simulink model "DC_motor"  (R2021b)
settings: Solver=VariableStepAuto  StartTime=0.0  StopTime=10.0  RelTol=1e-3
values from neighbouring files (symbols this model uses):
  Cmax = 0.66    [DC_moteur.sldd]
  Imax = 10.0    [DC_moteur.sldd]
  Ke = 0.041    [DC_moteur.sldd]
  Kt = 0.06    [DC_moteur.sldd]
  L = 0.00074    [DC_moteur.sldd]
  N1 = 4.25    [DC_moteur.sldd]
  R = 0.3    [DC_moteur.sldd]
  SigI = 0.05    [DC_moteur.sldd]
  Tech_Current = 0.01    [DC_moteur.sldd]
  vf_mot = 0.0    [DC_moteur.sldd]
libraries: simulink x1
settings Model: DataDictionary=DC_moteur.sldd  EnableAccessToBaseWorkspace=off  Creator=hugo  LastModifiedBy=hugo
settings SolverCC: ZeroCrossAlgorithm=Adaptive  AlgebraicLoopSolver=TrustRegion
settings DataIOCC: ReturnWorkspaceOutputs=off
settings DebuggingCC: SFMachineParentedDataDiag=warning  ArithmeticOperatorsInVariantConditions=warning
settings ModelReferenceCC: ModelReferenceMinAlgLoopOccurrences=on
settings SFSimCC: SimUseLocalCustomCode=off  CustomCodeUndefinedFunction=UseInterfaceOnly
settings RTWCC: RTWUseLocalCustomCode=off

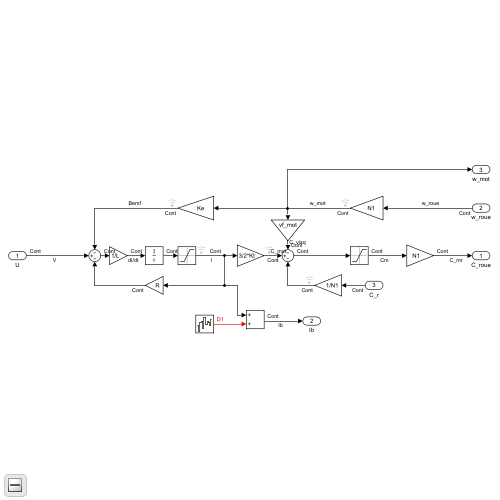
[thumbnail: Simulink's stored preview of the top-level diagram]
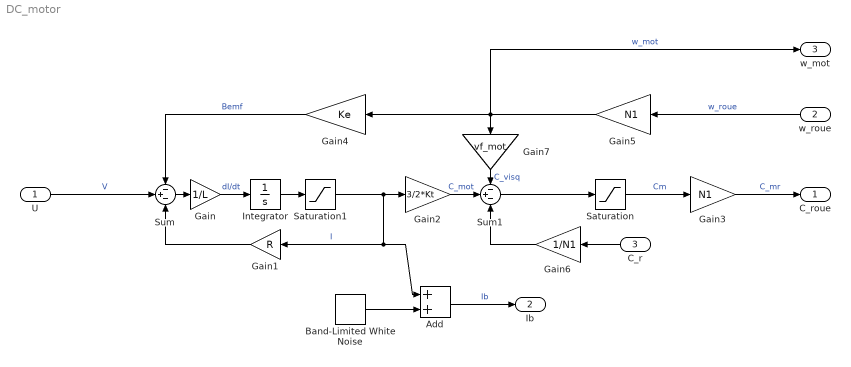
== system DC_motor ==
  U : Inport
  w_roue : Inport  Port=2
  C_r : Inport  Port=3
  Add : Sum
  Band-Limited White Noise : simulink/Sources/Band-Limited White Noise  Cov=(SigI)^2/(Tech_Current/2)  Ts=Tech_Current/2  seed=[23341]
  Gain : Gain  Gain=1/L
  Gain1 : Gain  Gain=R
  Gain2 : Gain  Gain=3/2*Kt
  Gain3 : Gain  Gain=N1
  Gain4 : Gain  Gain=Ke
  Gain5 : Gain  Gain=N1
  Gain6 : Gain  Gain=1/N1
  Gain7 : Gain  Gain=vf_mot
  Integrator : Integrator  ContinuousStateAttributes='Courant_Moteur'
  Saturation : Saturate  UpperLimit=Cmax  LowerLimit=-Cmax
  Saturation1 : Saturate  UpperLimit=Imax  LowerLimit=-Imax
  Sum : Sum  Inputs=-+-
  Sum1 : Sum  Inputs=-+-
  C_roue : Outport  VectorParamsAs1DForOutWhenUnconnected=off
  Ib : Outport  Port=2  VectorParamsAs1DForOutWhenUnconnected=off
  w_mot : Outport  Port=3
  wires:
  Band-Limited White Noise/1 -> Add/2
  Saturation/1 -> Gain3/1  "Cm"
  Gain6/1 -> Sum1/3
  Sum1/1 -> Saturation/1
  C_r/1 -> Gain6/1
  Gain5/1 -> w_mot/1, Gain4/1, Gain7/1  "w_mot"
  w_roue/1 -> Gain5/1  "w_roue"
  Add/1 -> Ib/1  "Ib"
  Gain/1 -> Integrator/1  "dI/dt"
  Sum/1 -> Gain/1
  Gain3/1 -> C_roue/1  "C_mr"
  Integrator/1 -> Saturation1/1
  Gain4/1 -> Sum/1  "Bemf"
  U/1 -> Sum/2  "V"
  Gain1/1 -> Sum/3
  Gain7/1 -> Sum1/1  "C_visq"
  Gain2/1 -> Sum1/2  "C_mot"
  Saturation1/1 -> Gain2/1, Gain1/1, Add/1  "I"
